simulink model "ExampleNavigationMessage"  (R2018b)
settings: Solver=FixedStepAuto  StartTime=0.0  StopTime=0  FixedStep=0.01  RelTol=1e-3
undefined symbols (not defined in the file): orientationRollPitchYaw, orientationYaw, positionEast, positionNED, positionNorth
libraries: InterModuleProtocol x5
settings Model: Creator=Scythe  LastModifiedBy=Scythe

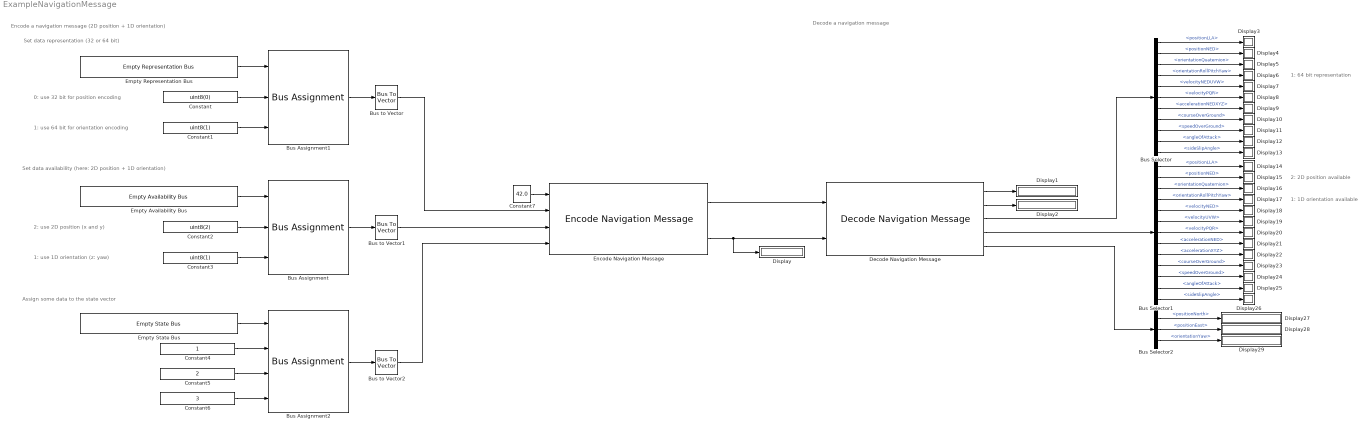
== system ExampleNavigationMessage ==
  note: Decode a navigation message
  note: Encode a navigation message (2D position + 1D orientation)
  note: Assign some data to the state vector
  note: Set data availability (here: 2D position + 1D orientation)
  note: Set data representation (32 or 64 bit)
  note: 0: use 32 bit for position encoding
  note: 1: use 64 bit for orientation encoding
  note: 2: use 2D position (x and y)
  note: 1: use 1D orientation (z: yaw)
  note: 1: 64 bit representation
  note: 2: 2D position available
  note: 1: 1D orientation available
  Bus Assignment : BusAssignment  AssignedSignals=positionNED,orientationRollPitchYaw
  Bus Assignment1 : BusAssignment  AssignedSignals=positionNED,orientationRollPitchYaw
  Bus Assignment2 : BusAssignment  AssignedSignals=positionNorth,positionEast,orientationYaw
  Bus Selector : BusSelector  OutputSignals=positionLLA,positionNED,orientationQuaternion,orientationRollPitchYaw,velocityNEDUVW,velocityPQR,accelerationNEDXYZ,courseOverGround,speedOverGround,angleOfAttack,sideSlipAngle
  Bus Selector1 : BusSelector  OutputSignals=positionLLA,positionNED,orientationQuaternion,orientationRollPitchYaw,velocityNED,velocityUVW,velocityPQR,accelerationNED,accelerationXYZ,courseOverGround,speedOverGround,angleOfAttack,sideSlipAngle
  Bus Selector2 : BusSelector  OutputSignals=positionNorth,positionEast,orientationYaw
  Bus to Vector : BusToVector
  Bus to Vector1 : BusToVector
  Bus to Vector2 : BusToVector
  Constant : Constant  Value=uint8(0)
  Constant1 : Constant  Value=uint8(1)
  Constant2 : Constant  Value=uint8(2)
  Constant3 : Constant  Value=uint8(1)
  Constant4 : Constant
  Constant5 : Constant  Value=2
  Constant6 : Constant  Value=3
  Constant7 : Constant  Value=42.0
  Decode Navigation Message : InterModuleProtocol/Decode Navigation Message
      settings: SourceProductName=Inter-Module Protocol
  Display{,1..29} (30 alike) : Display
  Empty Availability Bus : InterModuleProtocol/Empty Availability Bus
      settings: SourceProductName=Inter-Module Protocol
  Empty Representation Bus : InterModuleProtocol/Empty Representation Bus
      settings: SourceProductName=Inter-Module Protocol
  Empty State Bus : InterModuleProtocol/Empty State Bus
      settings: SourceProductName=Inter-Module Protocol
  Encode Navigation Message : InterModuleProtocol/Encode Navigation Message  outputBufferSize=268
      settings: SourceProductName=Inter-Module Protocol
  wires:
  Empty Availability Bus/1 -> Bus Assignment/1
  Empty Representation Bus/1 -> Bus Assignment1/1
  Constant/1 -> Bus Assignment1/2
  Constant1/1 -> Bus Assignment1/3
  Constant2/1 -> Bus Assignment/2
  Constant3/1 -> Bus Assignment/3
  Empty State Bus/1 -> Bus Assignment2/1
  Bus Assignment1/1 -> Bus to Vector/1
  Bus Assignment/1 -> Bus to Vector1/1
  Bus to Vector/1 -> Encode Navigation Message/2
  Bus to Vector1/1 -> Encode Navigation Message/3
  Bus to Vector2/1 -> Encode Navigation Message/4
  Bus Assignment2/1 -> Bus to Vector2/1
  Encode Navigation Message/1 -> Decode Navigation Message/1
  Encode Navigation Message/2 -> Decode Navigation Message/2, Display/1
  Constant4/1 -> Bus Assignment2/2
  Constant5/1 -> Bus Assignment2/3
  Constant6/1 -> Bus Assignment2/4
  Decode Navigation Message/1 -> Display1/1
  Decode Navigation Message/2 -> Display2/1
  Constant7/1 -> Encode Navigation Message/1
  Decode Navigation Message/3 -> Bus Selector/1
  Bus Selector/1 -> Display3/1  "<positionLLA>"
  Bus Selector/2 -> Display4/1  "<positionNED>"
  Bus Selector/3 -> Display5/1  "<orientationQuaternion>"
  Bus Selector/4 -> Display6/1  "<orientationRollPitchYaw>"
  Bus Selector/5 -> Display7/1  "<velocityNEDUVW>"
  Bus Selector/6 -> Display8/1  "<velocityPQR>"
  Bus Selector/8 -> Display10/1  "<courseOverGround>"
  Bus Selector/7 -> Display9/1  "<accelerationNEDXYZ>"
  Bus Selector/9 -> Display11/1  "<speedOverGround>"
  Bus Selector/10 -> Display12/1  "<angleOfAttack>"
  Bus Selector/11 -> Display13/1  "<sideSlipAngle>"
  Decode Navigation Message/4 -> Bus Selector1/1
  Bus Selector1/1 -> Display14/1  "<positionLLA>"
  Bus Selector1/2 -> Display15/1  "<positionNED>"
  Bus Selector1/3 -> Display16/1  "<orientationQuaternion>"
  Bus Selector1/4 -> Display17/1  "<orientationRollPitchYaw>"
  Bus Selector1/5 -> Display18/1  "<velocityNED>"
  Bus Selector1/6 -> Display19/1  "<velocityUVW>"
  Bus Selector1/7 -> Display20/1  "<velocityPQR>"
  Bus Selector1/8 -> Display21/1  "<accelerationNED>"
  Bus Selector1/9 -> Display22/1  "<accelerationXYZ>"
  Bus Selector1/10 -> Display23/1  "<courseOverGround>"
  Bus Selector1/11 -> Display24/1  "<speedOverGround>"
  Bus Selector1/12 -> Display25/1  "<angleOfAttack>"
  Bus Selector1/13 -> Display26/1  "<sideSlipAngle>"
  Decode Navigation Message/5 -> Bus Selector2/1
  Bus Selector2/1 -> Display27/1  "<positionNorth>"
  Bus Selector2/2 -> Display28/1  "<positionEast>"
  Bus Selector2/3 -> Display29/1  "<orientationYaw>"
